simulink model "ejercicio"  (Simulink 5.0)
settings: Solver=ode45  StartTime=0.0  StopTime=500  RelTol=1e-3
undefined symbols (not defined in the file): a, am, b, bm, Gama
settings Model: LastModifiedBy=Administrador

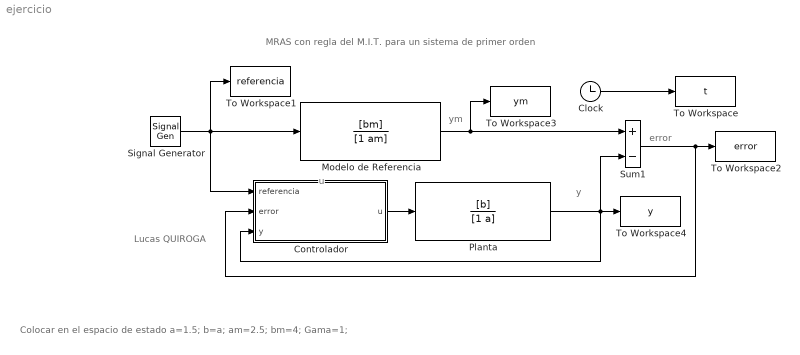
== system ejercicio ==
  note: y
  note: ym
  note: u
  note: error
  note: MRAS con regla del M.I.T. para un sistema de primer orden
  note: Lucas QUIROGA
  note: Colocar en el espacio de estado
      | a=1.5;
      | b=a;
      | am=2.5;
      | bm=4;
      | Gama=1;
  Clock : Clock
  Controlador : Subsystem
  Modelo de Referencia : TransferFcn  Numerator=[bm]  Denominator=[1 am]
  Planta : TransferFcn  Numerator=[b]  Denominator=[1 a]
  Signal Generator : SignalGenerator  WaveForm=square  Frequency=0.05
  Sum1 : Sum  Inputs=+-  SaturateOnIntegerOverflow=on
  To Workspace : ToWorkspace  VariableName=t  SampleTime=-1  SaveFormat=Array
  To Workspace1 : ToWorkspace  VariableName=referencia  SampleTime=-1  SaveFormat=Array
  To Workspace2 : ToWorkspace  VariableName=error  SampleTime=-1  SaveFormat=Array
  To Workspace3 : ToWorkspace  VariableName=ym  SampleTime=-1  SaveFormat=Array
  To Workspace4 : ToWorkspace  VariableName=y  SampleTime=-1  SaveFormat=Array
  wires:
  Controlador/1(u) -> Planta/1
  Signal Generator/1 -> Controlador/1(referencia), To Workspace1/1, Modelo de Referencia/1
  Modelo de Referencia/1 -> To Workspace3/1, Sum1/1
  Sum1/1 -> To Workspace2/1, Controlador/2(error)
  Clock/1 -> To Workspace/1
  Planta/1 -> Sum1/2, To Workspace4/1, Controlador/3(y)

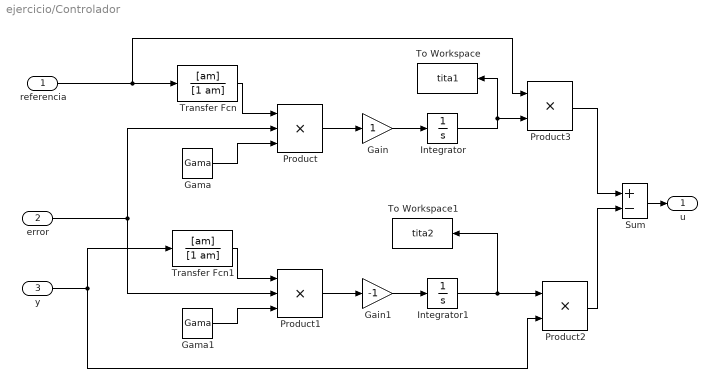
== system ejercicio/Controlador ==
  referencia : Inport
  error : Inport  Port=2
  y : Inport  Port=3
  Gain : Gain  SaturateOnIntegerOverflow=on
  Gain1 : Gain  Gain=-1  SaturateOnIntegerOverflow=on
  Gama : Constant  Value=Gama
  Gama1 : Constant  Value=Gama
  Integrator : Integrator
  Integrator1 : Integrator
  Product : Product  Inputs=3  SaturateOnIntegerOverflow=on
  Product1 : Product  Inputs=3  SaturateOnIntegerOverflow=on
  Product2 : Product  SaturateOnIntegerOverflow=on
  Product3 : Product  SaturateOnIntegerOverflow=on
  Sum : Sum  Inputs=+-  SaturateOnIntegerOverflow=on
  To Workspace : ToWorkspace  VariableName=tita1  SampleTime=-1  SaveFormat=Array
  To Workspace1 : ToWorkspace  VariableName=tita2  SampleTime=-1  SaveFormat=Array
  Transfer Fcn : TransferFcn  Numerator=[am]  Denominator=[1 am]
  Transfer Fcn1 : TransferFcn  Numerator=[am]  Denominator=[1 am]
  u : Outport
  wires:
  Gain/1 -> Integrator/1
  Product/1 -> Gain/1
  Transfer Fcn/1 -> Product/1
  Gama/1 -> Product/3
  Integrator/1 -> To Workspace/1, Product3/2
  Gain1/1 -> Integrator1/1
  Product1/1 -> Gain1/1
  Transfer Fcn1/1 -> Product1/1
  Gama1/1 -> Product1/3
  Integrator1/1 -> To Workspace1/1, Product2/1
  referencia/1 -> Product3/1, Transfer Fcn/1
  error/1 -> Product1/2, Product/2
  y/1 -> Product2/2, Transfer Fcn1/1
  Product2/1 -> Sum/2
  Product3/1 -> Sum/1
  Sum/1 -> u/1
